simulink model "FordFocus2013_DirectDrive_2016a"  (R2016a)
settings: Solver=FixedStepAuto  SolverMode=SingleTasking  StartTime=0.0  StopTime=len  FixedStep=1e-3  RelTol=1e-3
values from neighbouring files (symbols this model uses):
  logvars = 4    [runFocusValidation_WindsorMotor_DirectDrive.m]
undefined symbols (not defined in the file or in its folder): accessory_load, chassis, driver, enviro, ess, fd, motor, veh_init_speed, wheel
libraries: simulink x2
settings Model: SimulationMode=accelerator  Creator=leahe  LastModifiedBy=chris
settings SolverCC: ZeroCrossAlgorithm=Adaptive
settings DataIOCC: LimitDataPoints=on  SaveFormat=Array
settings OptimizationCC: BlockReduction=off  BooleanDataType=off  EfficientMapNaN2IntZero=off
settings DebuggingCC: SaveWithParameterizedLinksMsg=none  UnderspecifiedInitializationDetection=Classic  MergeDetectMultiDrivingBlocksExec=none  SignalResolutionControl=TryResolveAllWithWarning
settings HardwareCC: ProdBitPerPointer=32  ProdLargestAtomicFloat=None  ProdIntDivRoundTo=Undefined  ProdEndianess=Unspecified  ProdWordSize=32  ProdHWDeviceType=32-bit Generic  TargetBitPerPointer=64  TargetLongLongMode=on  TargetIntDivRoundTo=Zero  TargetEndianess=LittleEndian  TargetWordSize=64  TargetHWDeviceType=MATLAB Host  ProdEqTarget=off
settings ModelReferenceCC: PropagateSignalLabelsOutOfModel=off
settings CodeAppCC: MaxIdLength=128
settings GRTTargetCC: GeneratePreprocessorConditionals=Use local settings  CombineOutputUpdateFcns=off  GRTInterface=on
settings ConfigComp: CovSFcnEnable=off

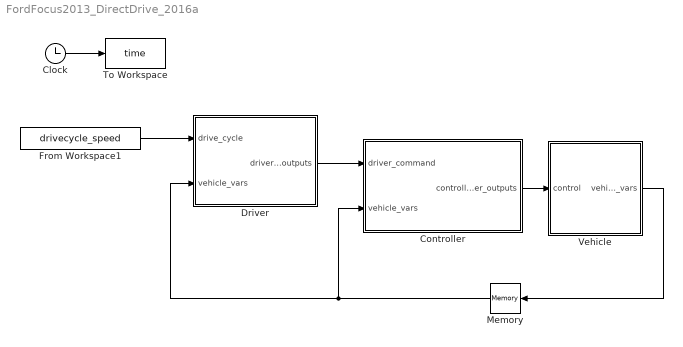
== system FordFocus2013_DirectDrive_2016a ==
  Clock : Clock
  Controller : Subsystem
  Driver : Subsystem
  From Workspace1 : FromWorkspace  VariableName=drivecycle_speed  SampleTime=0
  Memory : Memory
  To Workspace : ToWorkspace  VariableName=time  SampleTime=-1
      settings: Decimation=dec
  Vehicle : Subsystem
  wires:
  From Workspace1/1 -> Driver/1(drive_cycle)
  Memory/1 -> Driver/2(vehicle_vars), Controller/2(vehicle_vars)
  Controller/1(controller_outputs) -> Vehicle/1(control)
  Driver/1(driver_outputs) -> Controller/1(driver_command)
  Vehicle/1(vehicle_vars) -> Memory/1
  Clock/1 -> To Workspace/1

== system FordFocus2013_DirectDrive_2016a/Controller ==
  driver_command : Inport
  vehicle_vars : Inport  Port=2
  Bus Creator : BusCreator  Inputs=2
  Bus Selector : BusSelector  OutputSignals=trq_accel_dmd,trq_brk_dmd
  Bus Selector1 : BusSelector  OutputSignals=mot.mot_w,chas,ess1.ess_plant_volt_out
  Control Logic : Subsystem
  controller_outputs : Outport
  wires:
  driver_command/1 -> Bus Selector/1
  vehicle_vars/1 -> Bus Selector1/1
  Bus Creator/1 -> controller_outputs/1
  Bus Selector/1 -> Control Logic/1(driver_acceleration_cmd)  "<trq_accel_dmd>"
  Bus Selector/2 -> Control Logic/2(driver_brake_cmd)  "<trq_brk_dmd>"
  Control Logic/1(motor_trq_dmd) -> Bus Creator/1  "mot_trq_dmd"
  Control Logic/2(vehicle_wheel_dmd) -> Bus Creator/2  "whl_brk_trq_dmd"
  Bus Selector1/1 -> Control Logic/3(vehicle_motor_speed)  "<mot_w>"
  Bus Selector1/2 -> Control Logic/4(vehicle_chassis_speed)  "<chas>"
  Bus Selector1/3 -> Control Logic/5(ess2_voltage)  "<ess_plant_volt_out>"

== system FordFocus2013_DirectDrive_2016a/Driver ==
  drive_cycle : Inport
  vehicle_vars : Inport  Port=2
  Bus Creator1 : BusCreator  Inputs=3
  Bus Selector : BusSelector  OutputSignals=chas
  Plant : Subsystem
  Scope : Scope  NumInputPorts=2
  driver_outputs : Outport
  wires:
  drive_cycle/1 -> Scope/1, Plant/1(drive_cycle)
  Plant/1(driver_speed_dmd) -> Bus Creator1/1  "drv_lin_spd_dmd"
  vehicle_vars/1 -> Bus Selector/1
  Bus Selector/1 -> Scope/2, Plant/2(chassis_speed)  "<chas>"
  Bus Creator1/1 -> driver_outputs/1
  Plant/2(motor_torque_dmd) -> Bus Creator1/2  "trq_accel_dmd"
  Plant/3(wheel_brake_dmd) -> Bus Creator1/3  "trq_brk_dmd"

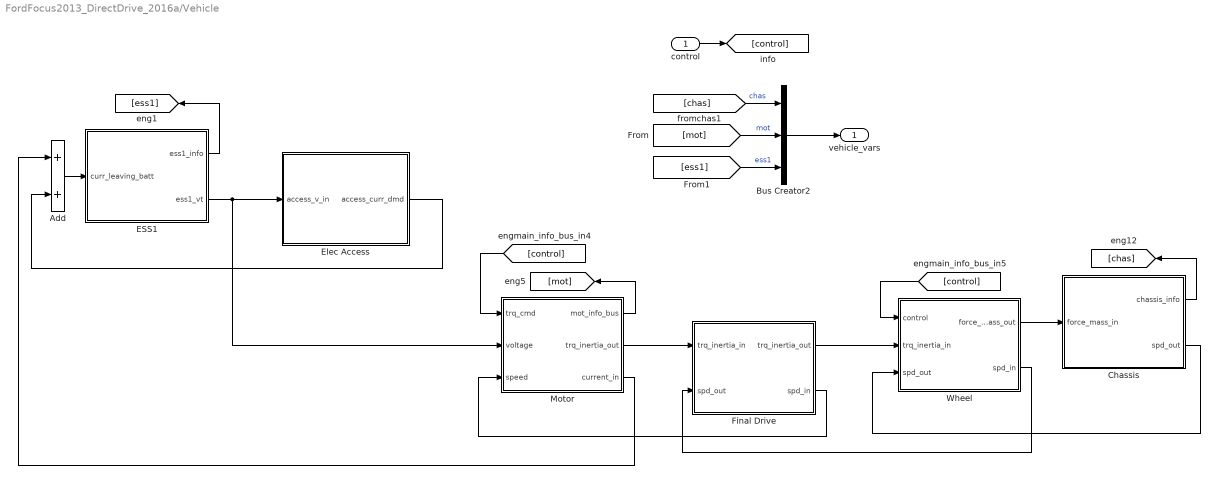
== system FordFocus2013_DirectDrive_2016a/Vehicle ==
  control : Inport
  Add : Sum
  Bus Creator2 : BusCreator  Inputs=3
  Chassis : Subsystem
  ESS1 : Subsystem
  Elec Access : Subsystem
  Final Drive : Subsystem
  Motor : Subsystem
  Wheel : Subsystem
  vehicle_vars : Outport
  wires:
  control/1 -> [control]
  Wheel/1(force_mass_out) -> Chassis/1(force_mass_in)
  Wheel/2(spd_in) -> Final Drive/2(spd_out)
  Chassis/2(spd_out) -> Wheel/3(spd_out)
  Final Drive/1(trq_inertia_out) -> Wheel/2(trq_inertia_in)
  [control] -> Wheel/1(control)
  Chassis/1(chassis_info) -> [chas]
  Bus Creator2/1 -> vehicle_vars/1
  [control] -> Motor/1(trq_cmd)
  Motor/2(trq_inertia_out) -> Final Drive/1(trq_inertia_in)
  Final Drive/2(spd_in) -> Motor/3(speed)
  Motor/1(mot_info_bus) -> [mot]
  Motor/3(current_in) -> Add/1
  [chas] -> Bus Creator2/1  "chas"
  [mot] -> Bus Creator2/2  "mot"
  Elec Access/1(access_curr_dmd) -> Add/2
  ESS1/2(ess1_vt) -> Motor/2(voltage), Elec Access/1(access_v_in)
  Add/1 -> ESS1/1(curr_leaving_batt)
  ESS1/1(ess1_info) -> [ess1]
  [ess1] -> Bus Creator2/3  "ess1"

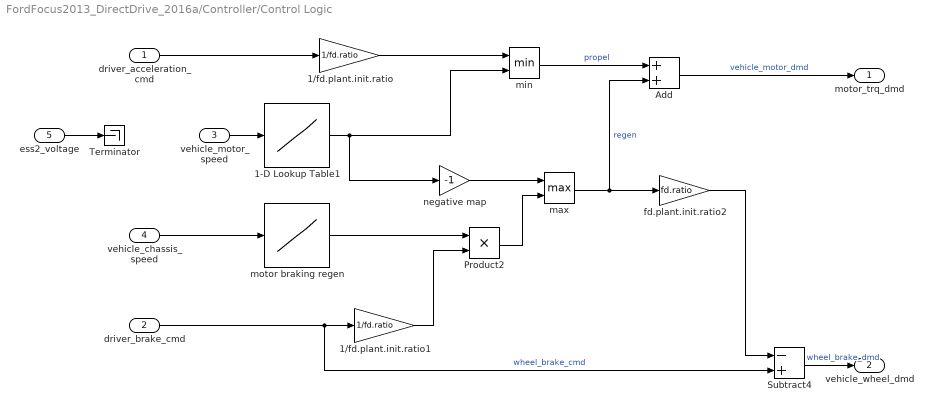
== system FordFocus2013_DirectDrive_2016a/Controller/Control Logic ==
  driver_acceleration_cmd : Inport
  driver_brake_cmd : Inport  Port=2
  vehicle_motor_speed : Inport  Port=3
  vehicle_chassis_speed : Inport  Port=4
  ess2_voltage : Inport  Port=5
  1-D Lookup Table1 : Lookup_n-D  NumberOfTableDimensions=1  BreakpointsForDimension1=motor.torquespeed_RPMidx  BreakpointsForDimension2=motor.torquespeed_RPMidx  IndexSearchMethod=Linear search  Table=motor.torquespeed_curveTOT  ExtrapMethod=Clip  UseLastTableValue=on  InternalRulePriority=Speed  RndMeth=Simplest  InputSameDT=on
  1/fd.plant.init.ratio : Gain  Gain=1/fd.ratio  SaturateOnIntegerOverflow=on  OutDataTypeStr=Inherit: Same as input  ParamDataTypeStr=Inherit: Same as input
  1/fd.plant.init.ratio1 : Gain  Gain=1/fd.ratio  SaturateOnIntegerOverflow=on  OutDataTypeStr=Inherit: Same as input  ParamDataTypeStr=Inherit: Same as input
  Add : Sum
  Product2 : Product
  Subtract4 : Sum  Inputs=-+
  Terminator : Terminator
  fd.plant.init.ratio2 : Gain  Gain=fd.ratio  SaturateOnIntegerOverflow=on  OutDataTypeStr=Inherit: Same as input  ParamDataTypeStr=Inherit: Same as input
  max : MinMax  Function=max  Inputs=2
  min : MinMax  Inputs=2
  motor braking regen : Lookup_n-D  NumberOfTableDimensions=1  BreakpointsForDimension1=motor.brake_idx  Table=motor.brake_map  InternalRulePriority=Speed  RndMeth=Simplest  InputSameDT=on
  negative map : Gain  Gain=-1  SaturateOnIntegerOverflow=on  OutDataTypeStr=Inherit: Same as input  ParamDataTypeStr=Inherit: Same as input
  motor_trq_dmd : Outport
  vehicle_wheel_dmd : Outport  Port=2
  wires:
  1/fd.plant.init.ratio/1 -> min/1
  1/fd.plant.init.ratio1/1 -> Product2/2
  Subtract4/1 -> vehicle_wheel_dmd/1  "wheel_brake_dmd"
  vehicle_chassis_speed/1 -> motor braking regen/1
  Product2/1 -> max/2
  vehicle_motor_speed/1 -> 1-D Lookup Table1/1
  driver_brake_cmd/1 -> Subtract4/2, 1/fd.plant.init.ratio1/1  "wheel_brake_cmd"
  driver_acceleration_cmd/1 -> 1/fd.plant.init.ratio/1
  min/1 -> Add/1  "propel"
  Add/1 -> motor_trq_dmd/1  "vehicle_motor_dmd"
  motor braking regen/1 -> Product2/1
  fd.plant.init.ratio2/1 -> Subtract4/1
  max/1 -> fd.plant.init.ratio2/1, Add/2  "regen"
  1-D Lookup Table1/1 -> negative map/1, min/2
  negative map/1 -> max/1
  ess2_voltage/1 -> Terminator/1

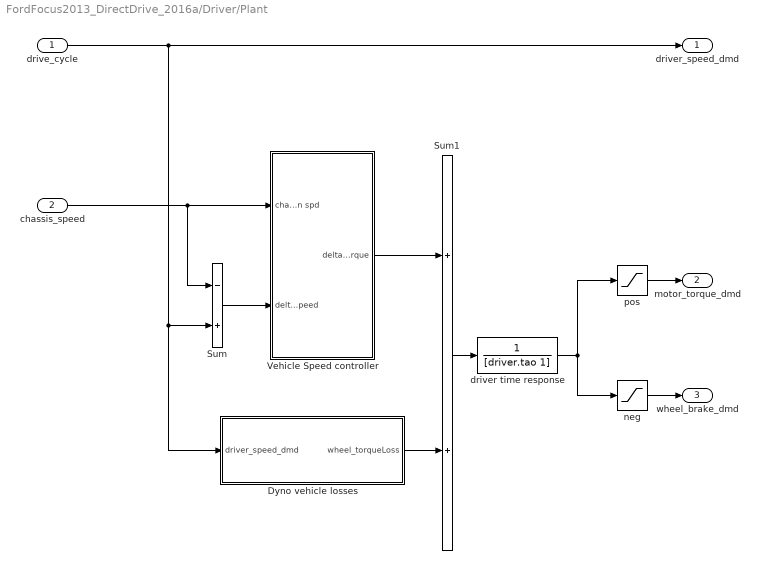
== system FordFocus2013_DirectDrive_2016a/Driver/Plant ==
  drive_cycle : Inport
  chassis_speed : Inport  Port=2
  Dyno vehicle losses : Subsystem
  Sum : Sum  Inputs=-+  SaturateOnIntegerOverflow=on  InputSameDT=on  OutDataTypeStr=Inherit: Same as first input
  Sum1 : Sum  Inputs=2  SaturateOnIntegerOverflow=on  InputSameDT=on  OutDataTypeStr=Inherit: Same as first input
  Vehicle Speed controller : Subsystem
  driver time response : TransferFcn  Denominator=[driver.tao 1]
  neg : Saturate  UpperLimit=0  LowerLimit=-inf
  pos : Saturate  UpperLimit=inf  LowerLimit=0
  driver_speed_dmd : Outport
  motor_torque_dmd : Outport  Port=2
  wheel_brake_dmd : Outport  Port=3
  wires:
  Vehicle Speed controller/1(delta torque) -> Sum1/1
  Dyno vehicle losses/1(wheel_torqueLoss) -> Sum1/2
  Sum/1 -> Vehicle Speed controller/2(delta speed)
  pos/1 -> motor_torque_dmd/1
  Sum1/1 -> driver time response/1
  neg/1 -> wheel_brake_dmd/1
  chassis_speed/1 -> Sum/1, Vehicle Speed controller/1(chas_lin spd)
  drive_cycle/1 -> Dyno vehicle losses/1(driver_speed_dmd), Sum/2, driver_speed_dmd/1
  driver time response/1 -> neg/1, pos/1

== system FordFocus2013_DirectDrive_2016a/Vehicle/Chassis ==
  force_mass_in : Inport
  From Workspace1 : FromWorkspace  VariableName=drivecycle_grade  SampleTime=0
  To Workspace : ToWorkspace  VariableName=chassis_speed  SampleTime=-1
      settings: Decimation=dec  Save2DSignal=2-D array (concatenate along first dimension)
  plant : Subsystem
  chassis_info : Outport
  spd_out : Outport  Port=2
  wires:
  plant/1(chas_lin_spd) -> spd_out/1, To Workspace/1, chassis_info/1
  force_mass_in/1 -> plant/2(chas_force_in chas_mass_in)
  From Workspace1/1 -> plant/1(Road grade)

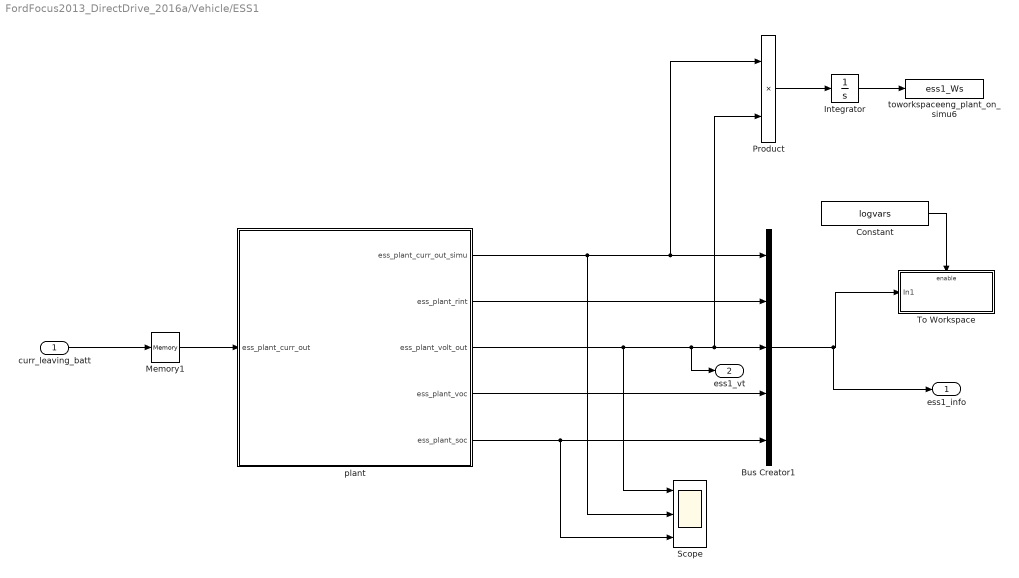
== system FordFocus2013_DirectDrive_2016a/Vehicle/ESS1 ==
  curr_leaving_batt : Inport
  Bus Creator1 : BusCreator  Inputs=5
  Constant : Constant  Value=logvars
  Integrator : Integrator
  Memory1 : Memory
  Product : Product
  Scope : Scope  NumInputPorts=3
  To Workspace : Subsystem  TreatAsAtomicUnit=on
  plant : Subsystem
  toworkspaceeng_plant_on_simu6 : ToWorkspace  VariableName=ess1_Ws  SampleTime=-1
      settings: Save2DSignal=2-D array (concatenate along first dimension)
  ess1_info : Outport
  ess1_vt : Outport  Port=2
  wires:
  Constant/1 -> To Workspace/Enable
  plant/4(ess_plant_voc) -> Bus Creator1/4
  plant/2(ess_plant_rint) -> Bus Creator1/2
  plant/1(ess_plant_curr_out_simu) -> Scope/2, Product/1, Bus Creator1/1
  curr_leaving_batt/1 -> Memory1/1
  Bus Creator1/1 -> ess1_info/1, To Workspace/1(In1)
  Memory1/1 -> plant/1(ess_plant_curr_out)
  plant/5(ess_plant_soc) -> Scope/3, Bus Creator1/5
  Product/1 -> Integrator/1
  Integrator/1 -> toworkspaceeng_plant_on_simu6/1
  plant/3(ess_plant_volt_out) -> Scope/1, ess1_vt/1, Product/2, Bus Creator1/3

== system FordFocus2013_DirectDrive_2016a/Vehicle/Elec Access ==
  access_v_in : Inport
  Electrical Power : Constant  Value=accessory_load
  Product : Product  Inputs=*/  SaturateOnIntegerOverflow=on  InputSameDT=on  OutDataTypeStr=Inherit: Same as first input
  Sum1 : Sum  SaturateOnIntegerOverflow=on  InputSameDT=on  OutDataTypeStr=Inherit: Same as first input
  eps : Constant  Value=eps
  access_curr_dmd : Outport
  wires:
  access_v_in/1 -> Sum1/1
  eps/1 -> Sum1/2
  Sum1/1 -> Product/2
  Electrical Power/1 -> Product/1
  Product/1 -> access_curr_dmd/1

== system FordFocus2013_DirectDrive_2016a/Vehicle/Final Drive ==
  trq_inertia_in : Inport
  spd_out : Inport  Port=2
  plant : Subsystem
  trq_inertia_out : Outport
  spd_in : Outport  Port=2
  wires:
  spd_out/1 -> plant/2(spd out)
  trq_inertia_in/1 -> plant/1(trq_inertia_in)
  plant/1(fd_trq_inertia_out) -> trq_inertia_out/1
  plant/2(fd_spd_in) -> spd_in/1

== system FordFocus2013_DirectDrive_2016a/Vehicle/Motor ==
  trq_cmd : Inport
  voltage : Inport  Port=2
  speed : Inport  Port=3
  Bus Creator : BusCreator  Inputs=3
  Bus Selector : BusSelector  OutputSignals=mot_trq_dmd
  motor : Subsystem
  mot_info_bus : Outport
  trq_inertia_out : Outport  Port=2
  current_in : Outport  Port=3
  wires:
  trq_cmd/1 -> Bus Selector/1
  voltage/1 -> motor/2(voltage)
  speed/1 -> motor/3(spd)
  motor/2(mot_current_in) -> Bus Creator/2, current_in/1
  motor/1(mot_trq_out mot_inertia_out) -> trq_inertia_out/1
  Bus Selector/1 -> motor/1(command_Nm)  "<mot_trq_dmd>"
  Bus Creator/1 -> mot_info_bus/1
  motor/4(motor_v_in) -> Bus Creator/3
  motor/3("speed out ") -> Bus Creator/1

== system FordFocus2013_DirectDrive_2016a/Vehicle/Wheel ==
  control : Inport
  trq_inertia_in : Inport  Port=2
  spd_out : Inport  Port=3
  Bus Selector : BusSelector  OutputSignals=whl_brk_trq_dmd
  From Workspace1 : FromWorkspace  VariableName=drivecycle_grade  SampleTime=0
  plant : Subsystem
  force_mass_out : Outport
  spd_in : Outport  Port=2
  wires:
  spd_out/1 -> plant/4(whl_spd)
  trq_inertia_in/1 -> plant/3(whl_trq_in whl_inertia_in)
  plant/2(whl_spd_in) -> spd_in/1
  plant/1(whl_force_out whl_mass_out) -> force_mass_out/1
  From Workspace1/1 -> plant/2(grade)
  control/1 -> Bus Selector/1
  Bus Selector/1 -> plant/1(brake trq dmd)  "<whl_brk_trq_dmd>"

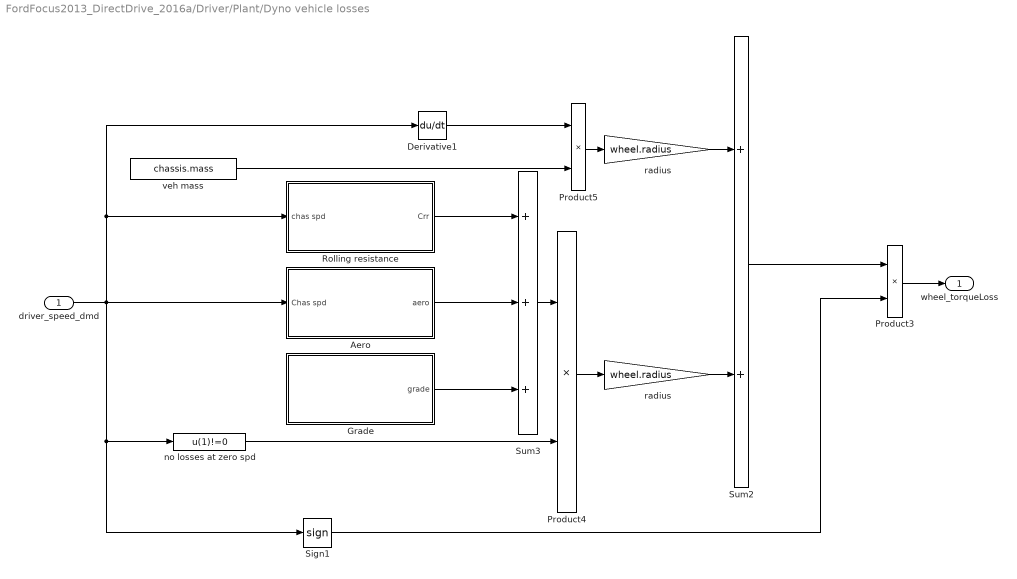
== system FordFocus2013_DirectDrive_2016a/Driver/Plant/Dyno vehicle losses ==
  driver_speed_dmd : Inport
  Aero : Subsystem
  Derivative1 : Derivative
  Grade : Subsystem
  Product3 : Product  SaturateOnIntegerOverflow=on  InputSameDT=on  OutDataTypeStr=Inherit: Same as first input
  Product4 : Product  SaturateOnIntegerOverflow=on  InputSameDT=on  OutDataTypeStr=Inherit: Same as first input
  Product5 : Product  SaturateOnIntegerOverflow=on  InputSameDT=on  OutDataTypeStr=Inherit: Same as first input
  Rolling resistance : Subsystem
  Sign1 : Signum
  Sum2 : Sum  Inputs=2  SaturateOnIntegerOverflow=on  InputSameDT=on  OutDataTypeStr=Inherit: Same as first input
  Sum3 : Sum  Inputs=3  SaturateOnIntegerOverflow=on  InputSameDT=on  OutDataTypeStr=Inherit: Same as first input
  no losses at zero spd : Fcn  Expr=u(1)!=0
  radius : Gain  Gain=wheel.radius  SaturateOnIntegerOverflow=on  OutDataTypeStr=Inherit: Same as input  ParamDataTypeStr=Inherit: Same as input
  "radius " : Gain  Gain=wheel.radius  SaturateOnIntegerOverflow=on  OutDataTypeStr=Inherit: Same as input  ParamDataTypeStr=Inherit: Same as input
  veh mass : Constant  Value=chassis.mass
  wheel_torqueLoss : Outport
  wires:
  "radius "/1 -> Sum2/2
  radius/1 -> Sum2/1
  no losses at zero spd/1 -> Product4/2
  Sum3/1 -> Product4/1
  Sign1/1 -> Product3/2
  veh mass/1 -> Product5/2
  Derivative1/1 -> Product5/1
  Product3/1 -> wheel_torqueLoss/1
  Sum2/1 -> Product3/1
  Product4/1 -> "radius "/1
  Product5/1 -> radius/1
  driver_speed_dmd/1 -> Sign1/1, no losses at zero spd/1, Aero/1(Chas spd), Derivative1/1, Rolling resistance/1(chas spd)
  Grade/1(grade) -> Sum3/3
  Aero/1(aero) -> Sum3/2
  Rolling resistance/1(Crr) -> Sum3/1

== system FordFocus2013_DirectDrive_2016a/Driver/Plant/Vehicle Speed controller ==
  chas_lin spd : Inport
  delta speed : Inport  Port=2  OutDataTypeStr=double
  "  1" : RelationalOperator  Operator=<  InputSameDT=on
  PID Controller : simulink/Continuous/PID Controller  Controller=PID  TimeDomain=Continuous-time  SampleTime=-1  IntegratorMethod=Forward Euler  FilterMethod=Forward Euler  Form=Parallel  UseFilter=on  ControllerParametersSource=internal  P=driver.p  I=driver.i  D=0  N=100  InitialConditionSource=internal  InitialConditionForIntegrator=0  InitialConditionForFilter=0  ExternalReset=either  LimitOutput=off  UpperSaturationLimit=inf  LowerSaturationLimit=-inf  LinearizeAsGain=on  AntiWindupMode=none  Kb=1  TrackingMode=off  Kt=1  PParamMin=[]  PParamMax=[]  IParamMin=[]  IParamMax=[]  DParamMin=[]  DParamMax=[]  NParamMin=[]  NParamMax=[]  KbParamMin=[]  KbParamMax=[]  KtParamMin=[]  KtParamMax=[]  POutMin=[]  POutMax=[]  IOutMin=[]  IOutMax=[]  DOutMin=[]  DOutMax=[]  NOutMin=[]  NOutMax=[]  KbOutMin=[]  KbOutMax=[]  KtOutMin=[]  KtOutMax=[]  IntegratorOutMin=[]  IntegratorOutMax=[]  FilterOutMin=[]  FilterOutMax=[]  SumOutMin=[]  SumOutMax=[]  SumI1OutMin=[]  SumI1OutMax=[]  SumI2OutMin=[]  SumI2OutMax=[]  SumI3OutMin=[]  SumI3OutMax=[]  SumDOutMin=[]  SumDOutMax=[]  SaturationOutMin=[]  SaturationOutMax=[]  IntegratorContinuousStateAttributes=''  IntegratorStateMustResolveToSignalObject=off  IntegratorRTWStateStorageClass=Auto  FilterContinuousStateAttributes=''  FilterStateMustResolveToSignalObject=off  FilterRTWStateStorageClass=Auto  DifferentiatorICPrevScaledInput=0  DifferentiatorOutMin=[]  DifferentiatorOutMax=[]
  "lin_spd_below_which_chas_stopped " : Constant  Value=driver.carStopped
  delta torque : Outport
  wires:
  PID Controller/1 -> delta torque/1
  chas_lin spd/1 -> "  1"/1
  "lin_spd_below_which_chas_stopped "/1 -> "  1"/2
  delta speed/1 -> PID Controller/1
  "  1"/1 -> PID Controller/2

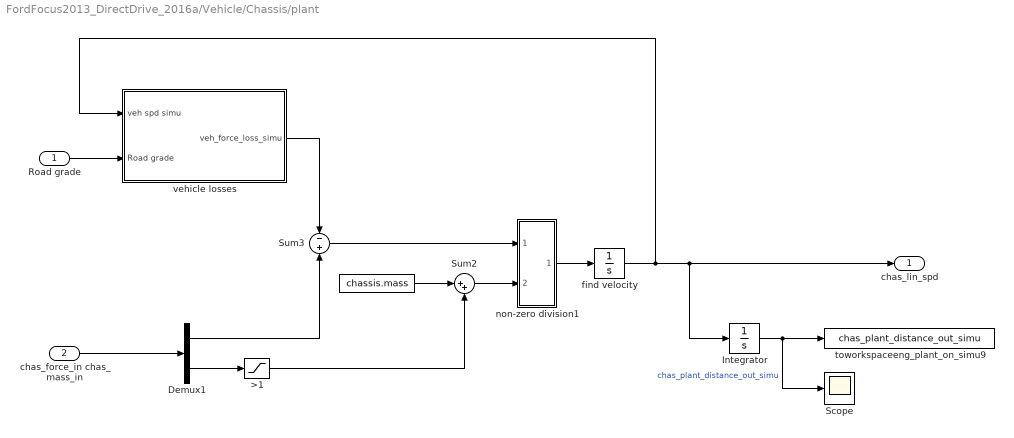
== system FordFocus2013_DirectDrive_2016a/Vehicle/Chassis/plant ==
  Road grade : Inport
  chas_force_in chas_mass_in : Inport  Port=2
  " " : Constant  Value=chassis.mass
  >1 : Saturate  UpperLimit=inf  LowerLimit=0
  Demux1 : Demux  Outputs=2
  Integrator : Integrator
  Scope : Scope
  Sum2 : Sum  Inputs=|++  SaturateOnIntegerOverflow=on  InputSameDT=on  OutDataTypeStr=Inherit: Same as first input
  Sum3 : Sum  Inputs=-+  SaturateOnIntegerOverflow=on  InputSameDT=on  OutDataTypeStr=Inherit: Same as first input
  find velocity : Integrator  InitialCondition=veh_init_speed  LimitOutput=on  LowerSaturationLimit=0
  non-zero division1 : Subsystem
      mask Display: disp('divider \n I1/I2')
  toworkspaceeng_plant_on_simu9 : ToWorkspace  VariableName=chas_plant_distance_out_simu  SampleTime=-1
      settings: Decimation=dec
  vehicle losses : Subsystem
  chas_lin_spd : Outport
  wires:
  Integrator/1 -> Scope/1, toworkspaceeng_plant_on_simu9/1  "chas_plant_distance_out_simu"
  " "/1 -> Sum2/1
  Road grade/1 -> vehicle losses/2(Road grade)
  find velocity/1 -> vehicle losses/1(veh spd simu), chas_lin_spd/1, Integrator/1
  non-zero division1/1(Out1) -> find velocity/1
  Sum3/1 -> non-zero division1/1(In1)
  Sum2/1 -> non-zero division1/2(In2)
  >1/1 -> Sum2/2
  Demux1/2 -> >1/1
  Demux1/1 -> Sum3/2
  chas_force_in chas_mass_in/1 -> Demux1/1
  vehicle losses/1(veh_force_loss_simu) -> Sum3/1

== system FordFocus2013_DirectDrive_2016a/Vehicle/ESS1/To Workspace ==
  In1 : Inport
  Enable : EnablePort
  Bus Selector : BusSelector  OutputSignals=ess_plant_curr_simu,ess_plant_rint,ess_plant_volt_out,ess_plant_voc,ess_plant_soc
  toworkspaceeng_plant_on_simu1 : ToWorkspace  VariableName=ess_i  SampleTime=-1
      settings: Decimation=dec
  toworkspaceeng_plant_on_simu2 : ToWorkspace  VariableName=ess_rint  SampleTime=-1
      settings: Decimation=dec
  toworkspaceeng_plant_on_simu3 : ToWorkspace  VariableName=ess_v  SampleTime=-1
      settings: Decimation=dec
  toworkspaceeng_plant_on_simu4 : ToWorkspace  VariableName=ess_voc  SampleTime=-1
      settings: Decimation=dec
  toworkspaceeng_plant_on_simu5 : ToWorkspace  VariableName=ess_soc  SampleTime=-1
      settings: Decimation=dec
  wires:
  Bus Selector/5 -> toworkspaceeng_plant_on_simu5/1  "<ess_plant_soc>"
  Bus Selector/4 -> toworkspaceeng_plant_on_simu4/1  "<ess_plant_voc>"
  Bus Selector/3 -> toworkspaceeng_plant_on_simu3/1  "<ess_plant_volt_out>"
  Bus Selector/2 -> toworkspaceeng_plant_on_simu2/1  "<ess_plant_rint>"
  Bus Selector/1 -> toworkspaceeng_plant_on_simu1/1  "<ess_plant_curr_simu>"
  In1/1 -> Bus Selector/1

== system FordFocus2013_DirectDrive_2016a/Vehicle/ESS1/plant ==
  ess_plant_curr_out : Inport
  Relational Operator : RelationalOperator  Operator=<  OutDataTypeStr=boolean
  Stop Simulation : Stop
  ess_plant_soc_calculation : Subsystem
  ess_plant_volt_calculation : Subsystem
  soc_min : Constant  Value=ess.soc_min
  ess_plant_curr_out_simu : Outport
  ess_plant_rint : Outport  Port=2
  ess_plant_volt_out : Outport  Port=3
  ess_plant_voc : Outport  Port=4
  ess_plant_soc : Outport  Port=5
  wires:
  ess_plant_curr_out/1 -> ess_plant_soc_calculation/1(ess_plant_curr_out), ess_plant_volt_calculation/2(Current), ess_plant_curr_out_simu/1  "ess_plant_curr_simu"
  ess_plant_volt_calculation/3(Rint) -> ess_plant_rint/1  "ess_plant_rint"
  ess_plant_volt_calculation/1(Voc) -> ess_plant_voc/1  "ess_plant_voc"
  ess_plant_volt_calculation/2(volt) -> ess_plant_volt_out/1  "ess_plant_volt_out"
  ess_plant_soc_calculation/1(ess_plant_soc) -> ess_plant_volt_calculation/1(SOC (prev)), Relational Operator/1, ess_plant_soc/1  "ess_plant_soc"
  soc_min/1 -> Relational Operator/2
  Relational Operator/1 -> Stop Simulation/1

== system FordFocus2013_DirectDrive_2016a/Vehicle/Final Drive/plant ==
  trq_inertia_in : Inport
  spd out : Inport  Port=2
  Demux : Demux  Outputs=2
  Inertia calculation : Subsystem
  Mux1 : Mux  Inputs=2
  Speed calculation : Subsystem
  Torque calculation : Subsystem
  fd_trq_inertia_out : Outport
  fd_spd_in : Outport  Port=2
  wires:
  spd out/1 -> Speed calculation/1(spd out)
  Torque calculation/1(trq out) -> Mux1/1  "fd_trq_out_simu"
  Demux/1 -> Torque calculation/2(trq in)
  Inertia calculation/1(inertia out) -> Mux1/2  "fd_inertia_out_simu"
  Demux/2 -> Inertia calculation/1(inertia in)
  Speed calculation/1(spd in) -> Torque calculation/1(spd in), fd_spd_in/1
  Mux1/1 -> fd_trq_inertia_out/1
  trq_inertia_in/1 -> Demux/1

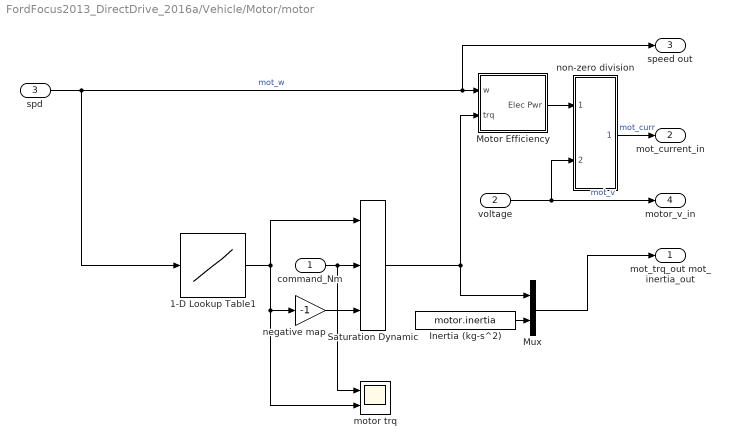
== system FordFocus2013_DirectDrive_2016a/Vehicle/Motor/motor ==
  command_Nm : Inport
  voltage : Inport  Port=2
  spd : Inport  Port=3
  1-D Lookup Table1 : Lookup_n-D  NumberOfTableDimensions=1  BreakpointsForDimension1=motor.torquespeed_RPMidx  BreakpointsForDimension2=motor.torquespeed_RPMidx  IndexSearchMethod=Linear search  Table=motor.torquespeed_curveTOT  ExtrapMethod=Clip  UseLastTableValue=on  InternalRulePriority=Speed  RndMeth=Simplest  InputSameDT=on
  Inertia (kg-s^2) : Constant  Value=motor.inertia
  Motor Efficiency : Subsystem
  Mux : Mux  Inputs=2
  Saturation Dynamic : simulink/Discontinuities/Saturation Dynamic  OutMin=[]  OutMax=[]  OutDataTypeStr=Inherit: Same as second input  OutDataType=fixdt(1, 16)  OutScaling=2^-10  DoSatur=off
  motor trq : Scope  NumInputPorts=2
  negative map : Gain  Gain=-1
  non-zero division : Subsystem
      mask Display: disp('divider \n I1/I2')
  mot_trq_out mot_inertia_out : Outport
  mot_current_in : Outport  Port=2
  "speed out " : Outport  Port=3
  motor_v_in : Outport  Port=4
  wires:
  non-zero division/1(Out1) -> mot_current_in/1  "mot_curr"
  Mux/1 -> mot_trq_out mot_inertia_out/1
  Inertia (kg-s^2)/1 -> Mux/2
  Saturation Dynamic/1 -> Motor Efficiency/2(trq), Mux/1
  Motor Efficiency/1(Elec Pwr) -> non-zero division/1(In1)
  negative map/1 -> Saturation Dynamic/3
  command_Nm/1 -> Saturation Dynamic/2, motor trq/1
  spd/1 -> 1-D Lookup Table1/1, "speed out "/1, Motor Efficiency/1(w)  "mot_w"
  1-D Lookup Table1/1 -> motor trq/2, negative map/1, Saturation Dynamic/1
  voltage/1 -> non-zero division/2(In2), motor_v_in/1  "mot_v"

== system FordFocus2013_DirectDrive_2016a/Vehicle/Wheel/plant ==
  brake trq dmd : Inport
  grade : Inport  Port=2
  whl_trq_in whl_inertia_in : Inport  Port=3
  whl_spd : Inport  Port=4
  "1\\radius " : Gain  Gain=1/wheel.radius  SaturateOnIntegerOverflow=on  OutDataTypeStr=Inherit: Same as input  ParamDataTypeStr=Inherit: Same as input
  Demux : Demux  Outputs=2
  Force calculation : Subsystem
  Mass calculation : Subsystem
  Mux1 : Mux  Inputs=2
  whl_force_out whl_mass_out : Outport
  whl_spd_in : Outport  Port=2
  wires:
  grade/1 -> Force calculation/2(grade)
  Mux1/1 -> whl_force_out whl_mass_out/1
  brake trq dmd/1 -> Force calculation/3(brake trq dmd)
  whl_trq_in whl_inertia_in/1 -> Demux/1
  whl_spd/1 -> Force calculation/1(whl_spd), "1\\radius "/1
  Demux/2 -> Mass calculation/1(inertia in)
  Demux/1 -> Force calculation/4(trq in)
  Mass calculation/1(Mass) -> Mux1/2  "whl_mass_out_simu"
  "1\\radius "/1 -> whl_spd_in/1
  Force calculation/1(force) -> Mux1/1  "whl_force_out_simu"

== system FordFocus2013_DirectDrive_2016a/Driver/Plant/Dyno vehicle losses/Aero ==
  Chas spd : Inport
  Gain : Gain  Gain=0.5
  Product2 : Product  Inputs=5  SaturateOnIntegerOverflow=on  InputSameDT=on  OutDataTypeStr=Inherit: Same as first input
  veh mass7 : Constant  Value=enviro.dens_air
  veh mass8 : Constant  Value=chassis.cd
  veh mass9 : Constant  Value=chassis.area
  aero : Outport
  wires:
  Product2/1 -> Gain/1
  veh mass7/1 -> Product2/3
  veh mass8/1 -> Product2/4
  veh mass9/1 -> Product2/5
  Chas spd/1 -> Product2/2, Product2/1
  Gain/1 -> aero/1  "Drag Force"

== system FordFocus2013_DirectDrive_2016a/Driver/Plant/Dyno vehicle losses/Grade ==
  From Workspace1 : FromWorkspace  VariableName=drivecycle_grade  SampleTime=0
  Product1 : Product  Inputs=3  SaturateOnIntegerOverflow=on  InputSameDT=on  OutDataTypeStr=Inherit: Same as first input
  Trigonometric Function1 : Trigonometry
  veh mass1 : Constant  Value=enviro.gravity
  veh mass2 : Constant  Value=chassis.mass
  grade : Outport
  wires:
  veh mass2/1 -> Product1/2
  From Workspace1/1 -> Trigonometric Function1/1
  Trigonometric Function1/1 -> Product1/1
  veh mass1/1 -> Product1/3
  Product1/1 -> grade/1  "Grade Force"

== system FordFocus2013_DirectDrive_2016a/Driver/Plant/Dyno vehicle losses/Rolling resistance ==
  chas spd : Inport
  From Workspace2 : FromWorkspace  VariableName=drivecycle_grade  SampleTime=0
  Product7 : Product  SaturateOnIntegerOverflow=on  InputSameDT=on  OutDataTypeStr=Inherit: Same as first input
  Product8 : Product  Inputs=4  SaturateOnIntegerOverflow=on  InputSameDT=on  OutDataTypeStr=Inherit: Same as first input
  Sum1 : Sum  Inputs=2  SaturateOnIntegerOverflow=on  InputSameDT=on  OutDataTypeStr=Inherit: Same as first input
  Trigonometric Function2 : Trigonometry  Operator=cos
  veh mass : Constant  Value=chassis.mass
  veh mass4 : Constant  Value=wheel.u2
  veh mass5 : Constant  Value=wheel.u1
  veh mass6 : Constant  Value=enviro.gravity
  Crr : Outport
  wires:
  From Workspace2/1 -> Trigonometric Function2/1
  veh mass4/1 -> Product7/2
  veh mass5/1 -> Sum1/2
  Product7/1 -> Sum1/1
  Sum1/1 -> Product8/2
  veh mass6/1 -> Product8/3
  Trigonometric Function2/1 -> Product8/1
  veh mass/1 -> Product8/4
  chas spd/1 -> Product7/1
  Product8/1 -> Crr/1  "Rolling resistance"

== system FordFocus2013_DirectDrive_2016a/Vehicle/Chassis/plant/non-zero division1 ==
  note: (u[2]==0) is true then returns 1, thus (u[2]+(u[2]==0)) is equal to 0+1=1
  note: if u[2] == 0, then output == 0:
  note: (u[2]!=0) is false then returns 0
  note: and finally, the expression is: (u[1] \ 1) * 0 = 0
  note: (u[2]==0) is false then returns 0, thus (u[2]+(u[2]==0)) is equal to u[2]+0=u[2]
  note: if u[2] != 0, then output == u[1]\u[2]:
  note: (u[2]!=0) is true then returns 1
  note: and finally, the expression is: (u[1] \ u[2]) * 1 = u[1] \ u[2]
  In1 : Inport
  In2 : Inport  Port=2
  Fcn : Fcn  Expr=u[1]/(u[2]+(u[2]==0))*(u[2]!=0)
  Mux : Mux  Inputs=2
  Out1 : Outport
  wires:
  Mux/1 -> Fcn/1
  In1/1 -> Mux/1
  Fcn/1 -> Out1/1
  In2/1 -> Mux/2

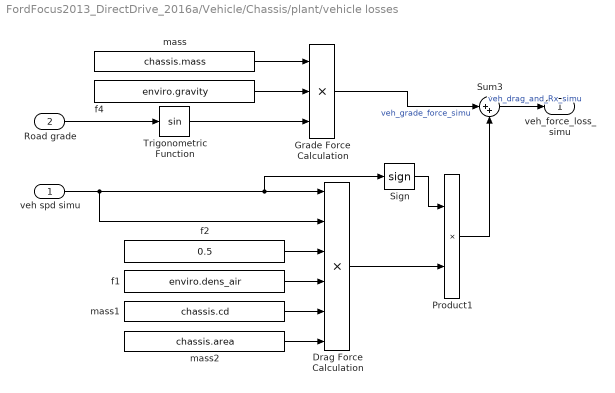
== system FordFocus2013_DirectDrive_2016a/Vehicle/Chassis/plant/vehicle losses ==
  veh spd simu : Inport
  Road grade : Inport  Port=2
  Drag Force Calculation : Product  Inputs=6  SaturateOnIntegerOverflow=on  InputSameDT=on  OutDataTypeStr=Inherit: Same as first input
  Grade Force Calculation : Product  Inputs=3  SaturateOnIntegerOverflow=on  InputSameDT=on  OutDataTypeStr=Inherit: Same as first input
  Product1 : Product  SaturateOnIntegerOverflow=on  InputSameDT=on  OutDataTypeStr=Inherit: Same as first input
  Sign : Signum
  Sum3 : Sum  Inputs=|++  SaturateOnIntegerOverflow=on  InputSameDT=on  OutDataTypeStr=Inherit: Same as first input
  Trigonometric Function : Trigonometry
  f1 : Constant  Value=enviro.dens_air
  f2 : Constant  Value=0.5
  f4 : Constant  Value=enviro.gravity
  mass : Constant  Value=chassis.mass
  mass1 : Constant  Value=chassis.cd
  mass2 : Constant  Value=chassis.area
  veh_force_loss_simu : Outport
  wires:
  f2/1 -> Drag Force Calculation/3
  mass2/1 -> Drag Force Calculation/6
  mass1/1 -> Drag Force Calculation/5
  f1/1 -> Drag Force Calculation/4
  Trigonometric Function/1 -> Grade Force Calculation/3
  f4/1 -> Grade Force Calculation/2
  mass/1 -> Grade Force Calculation/1
  Product1/1 -> Sum3/2
  Sign/1 -> Product1/1
  Road grade/1 -> Trigonometric Function/1
  Drag Force Calculation/1 -> Product1/2
  veh spd simu/1 -> Drag Force Calculation/1, Sign/1, Drag Force Calculation/2
  Grade Force Calculation/1 -> Sum3/1  "veh_grade_force_simu"
  Sum3/1 -> veh_force_loss_simu/1  "veh_drag_and_Rx_simu"

== system FordFocus2013_DirectDrive_2016a/Vehicle/ESS1/plant/ess_plant_soc_calculation ==
  ess_plant_curr_out : Inport
  (sec->hrs) : Gain  Gain=1/3600  SaturateOnIntegerOverflow=on  OutDataTypeStr=Inherit: Same as input  ParamDataTypeStr=Inherit: Same as input
  (sec->hrs)1 : Gain  Gain=-1  SaturateOnIntegerOverflow=on  OutDataTypeStr=Inherit: Same as input  ParamDataTypeStr=Inherit: Same as input
  Constant : Constant  Value=ess.soc_start
  Constant1 : Constant  Value=ess.cap
  Integrator : Integrator  InitialConditionSource=external
  Product : Product  RndMeth=Zero
  non-zero division1 : Subsystem
      mask Display: disp('divider \n I1/I2')
  ess_plant_soc : Outport
  wires:
  Constant1/1 -> non-zero division1/2(In2), Product/2
  non-zero division1/1(Out1) -> ess_plant_soc/1
  (sec->hrs)/1 -> (sec->hrs)1/1
  Integrator/1 -> non-zero division1/1(In1)
  Constant/1 -> Product/1
  Product/1 -> Integrator/2
  (sec->hrs)1/1 -> Integrator/1
  ess_plant_curr_out/1 -> (sec->hrs)/1

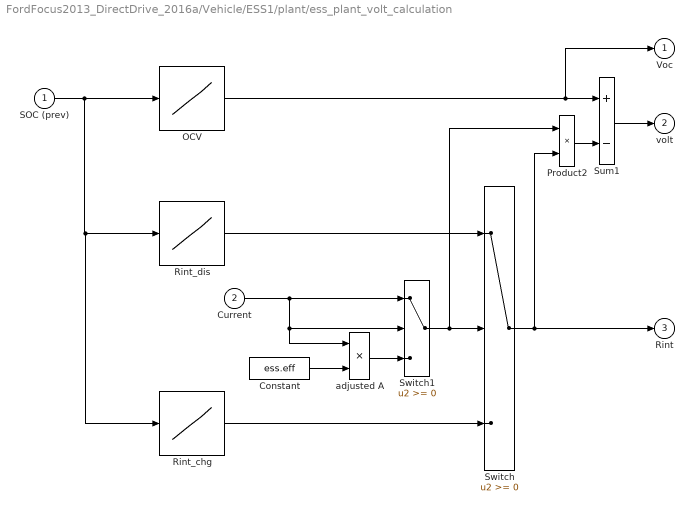
== system FordFocus2013_DirectDrive_2016a/Vehicle/ESS1/plant/ess_plant_volt_calculation ==
  SOC (prev) : Inport
  Current : Inport  Port=2
  Constant : Constant  Value=ess.eff
  OCV : Lookup_n-D  NumberOfTableDimensions=1  BreakpointsForDimension1=ess.idx_soc  BreakpointsForDimension2=ess.plant.init.voc.idx2_soc  Table=ess.ocv_map  ExtrapMethod=Clip  UseLastTableValue=on  RndMeth=Simplest  InputSameDT=on
  Product2 : Product  SaturateOnIntegerOverflow=on  InputSameDT=on  OutDataTypeStr=Inherit: Same as first input
  Rint_chg : Lookup_n-D  NumberOfTableDimensions=1  BreakpointsForDimension1=ess.rchg.idx_soc  BreakpointsForDimension2=ess.plant.init.rint_chg.idx2_soc  Table=ess.rchg_map  ExtrapMethod=Clip  UseLastTableValue=on  RndMeth=Simplest  InputSameDT=on
  Rint_dis : Lookup_n-D  NumberOfTableDimensions=1  BreakpointsForDimension1=ess.rdis.idx_soc  BreakpointsForDimension2=ess.plant.init.rint_dis.idx2_soc  Table=ess.rdis_map  ExtrapMethod=Clip  UseLastTableValue=on  RndMeth=Simplest  InputSameDT=on
  Sum1 : Sum  Inputs=+-  SaturateOnIntegerOverflow=on  InputSameDT=on  OutDataTypeStr=Inherit: Same as first input
  Switch : Switch  SaturateOnIntegerOverflow=on  InputSameDT=on
  Switch1 : Switch  SaturateOnIntegerOverflow=on  InputSameDT=on
  adjusted A : Product  SaturateOnIntegerOverflow=on  InputSameDT=on  OutDataTypeStr=Inherit: Same as first input
  Voc : Outport  InitialOutput=0
  volt : Outport  Port=2  InitialOutput=0
  Rint : Outport  Port=3  InitialOutput=0
  wires:
  Switch/1 -> Rint/1, Product2/2
  Switch1/1 -> Switch/2, Product2/1
  Rint_dis/1 -> Switch/1
  Rint_chg/1 -> Switch/3
  OCV/1 -> Sum1/1, Voc/1
  SOC (prev)/1 -> OCV/1, Rint_dis/1, Rint_chg/1
  Product2/1 -> Sum1/2
  Sum1/1 -> volt/1
  Constant/1 -> adjusted A/2
  Current/1 -> Switch1/1, Switch1/2, adjusted A/1
  adjusted A/1 -> Switch1/3

== system FordFocus2013_DirectDrive_2016a/Vehicle/Final Drive/plant/Inertia calculation ==
  inertia in : Inport
  " " : Constant  Value=fd.inert
  Sum3 : Sum  Inputs=|++  SaturateOnIntegerOverflow=on  InputSameDT=on  OutDataTypeStr=Inherit: Same as first input
  fd.plant.init.ratio : Gain  Gain=fd.ratio  SaturateOnIntegerOverflow=on  OutDataTypeStr=Inherit: Same as input  ParamDataTypeStr=Inherit: Same as input
  inertia out : Outport
  wires:
  inertia in/1 -> fd.plant.init.ratio/1
  fd.plant.init.ratio/1 -> Sum3/1
  " "/1 -> Sum3/2
  Sum3/1 -> inertia out/1

== system FordFocus2013_DirectDrive_2016a/Vehicle/Final Drive/plant/Speed calculation ==
  spd out : Inport
  " " : Gain  Gain=fd.ratio  SaturateOnIntegerOverflow=on  OutDataTypeStr=Inherit: Same as input  ParamDataTypeStr=Inherit: Same as input
  spd in : Outport
  wires:
  spd out/1 -> " "/1
  " "/1 -> spd in/1

== system FordFocus2013_DirectDrive_2016a/Vehicle/Final Drive/plant/Torque calculation ==
  spd in : Inport
  trq in : Inport  Port=2
  " " : Gain  Gain=fd.ratio  SaturateOnIntegerOverflow=on  OutDataTypeStr=Inherit: Same as input  ParamDataTypeStr=Inherit: Same as input
  Abs : Abs  SaturateOnIntegerOverflow=on
  Abs1 : Abs  SaturateOnIntegerOverflow=on
  Efficiency : Lookup_n-D  BreakpointsForDimension1=fd.torque  BreakpointsForDimension2=fd.speed  Table=fd.effmap  ExtrapMethod=Clip  UseLastTableValue=on  InternalRulePriority=Speed  RndMeth=Simplest  InputSameDT=on
  Product1 : Product
  Sign : Signum
  Switch : Switch  Criteria=u2 > Threshold
  non-zero division1 : Subsystem
      mask Display: disp('divider \n I1/I2')
  trq out : Outport
  wires:
  Abs/1 -> Efficiency/1
  Abs1/1 -> Efficiency/2
  spd in/1 -> Abs1/1
  trq in/1 -> Sign/1, " "/1, Abs/1
  " "/1 -> Product1/2, non-zero division1/1(In1)
  Sign/1 -> Switch/2
  Switch/1 -> trq out/1
  Efficiency/1 -> non-zero division1/2(In2), Product1/1
  Product1/1 -> Switch/1
  non-zero division1/1(Out1) -> Switch/3

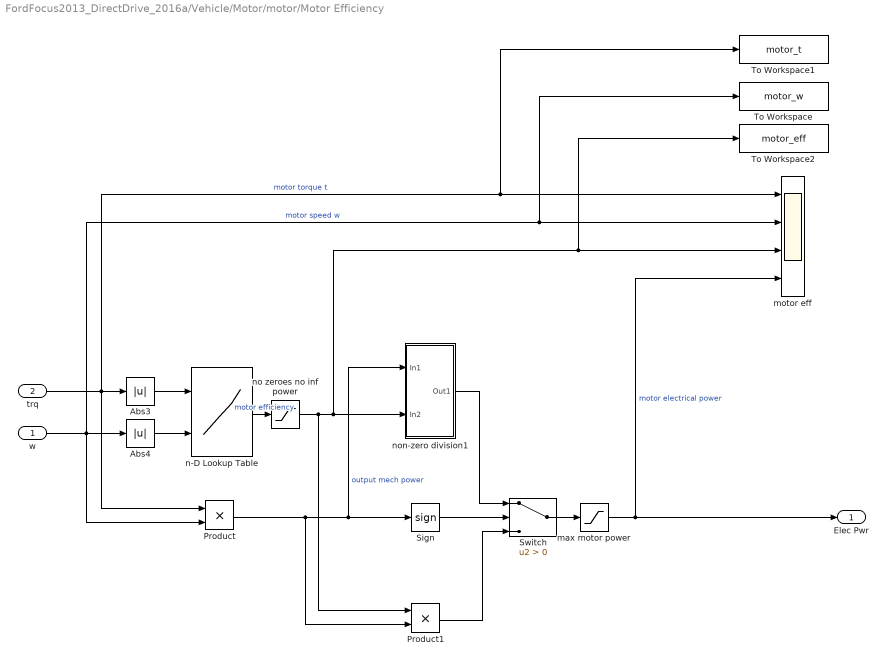
== system FordFocus2013_DirectDrive_2016a/Vehicle/Motor/motor/Motor Efficiency ==
  w : Inport
  trq : Inport  Port=2
  Abs3 : Abs
  Abs4 : Abs
  Product : Product
  Product1 : Product
  Sign : Signum
  Switch : Switch  Criteria=u2 > Threshold
  To Workspace : ToWorkspace  VariableName=motor_w  SampleTime=-1
      settings: Save2DSignal=2-D array (concatenate along first dimension)
  To Workspace1 : ToWorkspace  VariableName=motor_t  SampleTime=-1
      settings: Save2DSignal=2-D array (concatenate along first dimension)
  To Workspace2 : ToWorkspace  VariableName=motor_eff  SampleTime=-1
      settings: Save2DSignal=2-D array (concatenate along first dimension)
  max motor power : Saturate  UpperLimit=motor.prated  LowerLimit=-(motor.prated)  LinearizeAsGain=off
  motor eff : Scope  NumInputPorts=4
  n-D Lookup Table : Lookup_n-D  BreakpointsForDimension1=motor.spd_ind  BreakpointsForDimension2=motor.trq_ind  BreakpointsForDimension3=motor.vol_ind  IndexSearchMethod=Linear search  Table=motor.eff_map  ExtrapMethod=Clip  UseLastTableValue=on  InternalRulePriority=Speed  RndMeth=Simplest  InputSameDT=on
  no zeroes no inf power : Saturate  UpperLimit=1  LowerLimit=0.7  LinearizeAsGain=off
  non-zero division1 : Subsystem
      mask Display: disp('divider \n I1/I2')
  Elec Pwr : Outport
  wires:
  Sign/1 -> Switch/2
  non-zero division1/1(Out1) -> Switch/1
  Product1/1 -> Switch/3
  Product/1 -> Product1/2, non-zero division1/1(In1), Sign/1  "output mech power"
  Switch/1 -> max motor power/1
  max motor power/1 -> motor eff/4, Elec Pwr/1  "motor electrical power"
  w/1 -> Product/2, To Workspace/1, motor eff/2, Abs4/1  "motor speed w"
  trq/1 -> Product/1, motor eff/1, To Workspace1/1, Abs3/1  "motor torque t"
  n-D Lookup Table/1 -> no zeroes no inf power/1  "motor efficiency"
  Abs3/1 -> n-D Lookup Table/1
  Abs4/1 -> n-D Lookup Table/2
  no zeroes no inf power/1 -> Product1/1, To Workspace2/1, motor eff/3, non-zero division1/2(In2)

== system FordFocus2013_DirectDrive_2016a/Vehicle/Motor/motor/non-zero division ==
  note: original idea from Phil Sharer - ANL
      | original formula: u[1]\(u[2]+eps)*(u[2]!=0)
      | changes done by Gerald ZINI (dgey) - ANL (05\02\2001)
  note: (u[2]==0) is true then returns 1, thus (u[2]+(u[2]==0)) is equal to 0+1=1
  note: if u[2] == 0, then output == 0:
  note: (u[2]!=0) is false then returns 0
  note: and finally, the expression is: (u[1] \ 1) * 0 = 0
  note: (u[2]==0) is false then returns 0, thus (u[2]+(u[2]==0)) is equal to u[2]+0=u[2]
  note: if u[2] != 0, then output == u[1]\u[2]:
  note: (u[2]!=0) is true then returns 1
  note: and finally, the expression is: (u[1] \ u[2]) * 1 = u[1] \ u[2]
  In1 : Inport
  In2 : Inport  Port=2
  Fcn : Fcn  Expr=u[1]/(u[2]+(u[2]==0))*(u[2]!=0)
  Mux : Mux  Inputs=2
  Out1 : Outport
  wires:
  Mux/1 -> Fcn/1
  In1/1 -> Mux/1
  Fcn/1 -> Out1/1
  In2/1 -> Mux/2

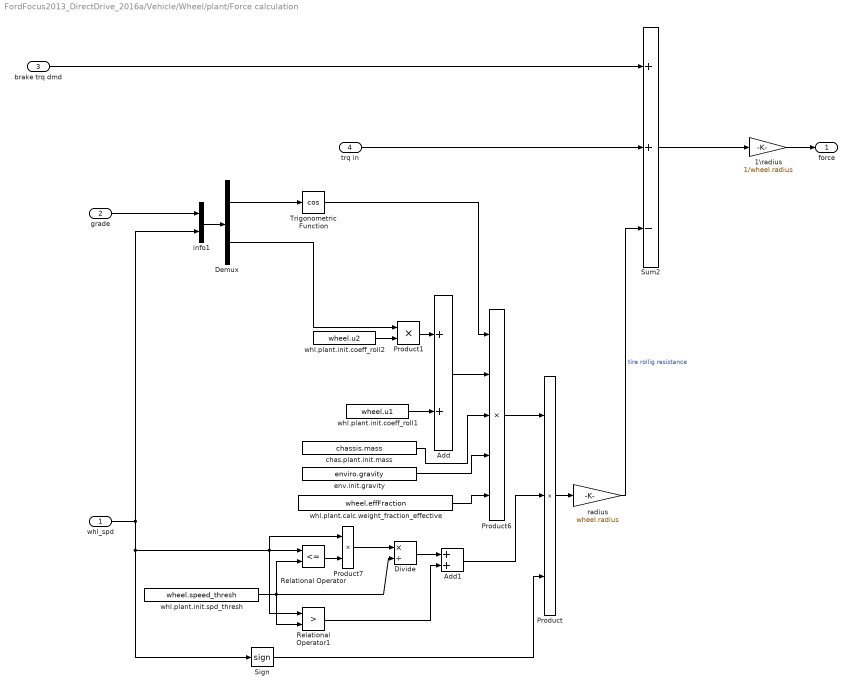
== system FordFocus2013_DirectDrive_2016a/Vehicle/Wheel/plant/Force calculation ==
  whl_spd : Inport
  grade : Inport  Port=2
  brake trq dmd : Inport  Port=3
  trq in : Inport  Port=4
  "1\\radius " : Gain  Gain=1/wheel.radius  SaturateOnIntegerOverflow=on  OutDataTypeStr=Inherit: Same as input  ParamDataTypeStr=Inherit: Same as input
  Add : Sum  Inputs=2
  Add1 : Sum
  Demux : Demux  Outputs=2
  Divide : Product  Inputs=*/
  Product : Product  Inputs=3  SaturateOnIntegerOverflow=on  InputSameDT=on  OutDataTypeStr=Inherit: Same as first input
  Product1 : Product  RndMeth=Zero
  Product6 : Product  Inputs=5  RndMeth=Zero
  Product7 : Product  RndMeth=Zero
  Relational Operator : RelationalOperator  Operator=<=  InputSameDT=on
  Relational Operator1 : RelationalOperator  Operator=>  InputSameDT=on
  Sign : Signum
  Sum2 : Sum  Inputs=++-  SaturateOnIntegerOverflow=on  InputSameDT=on  OutDataTypeStr=Inherit: Same as first input
  Trigonometric Function : Trigonometry  Operator=cos
  chas.plant.init.mass : Constant  Value=chassis.mass
  env.init.gravity : Constant  Value=enviro.gravity
  info1 : Mux  Inputs=2
  radius : Gain  Gain=wheel.radius  SaturateOnIntegerOverflow=on  OutDataTypeStr=Inherit: Same as input  ParamDataTypeStr=Inherit: Same as input
  whl.plant.calc.weight_fraction_effective : Constant  Value=wheel.effFraction
  whl.plant.init.coeff_roll1 : Constant  Value=wheel.u1
  whl.plant.init.coeff_roll2 : Constant  Value=wheel.u2
  whl.plant.init.spd_thresh : Constant  Value=wheel.speed_thresh
  force : Outport
  wires:
  Add1/1 -> Product/2
  Relational Operator1/1 -> Add1/2
  Divide/1 -> Add1/1
  Product7/1 -> Divide/1
  Relational Operator/1 -> Product7/2
  whl.plant.init.spd_thresh/1 -> Relational Operator1/2, Divide/2, Relational Operator/2
  Product6/1 -> Product/1
  Demux/1 -> Trigonometric Function/1
  Trigonometric Function/1 -> Product6/1
  whl.plant.calc.weight_fraction_effective/1 -> Product6/5
  env.init.gravity/1 -> Product6/4
  chas.plant.init.mass/1 -> Product6/3
  Add/1 -> Product6/2
  Product1/1 -> Add/1
  Demux/2 -> Product1/1
  whl.plant.init.coeff_roll2/1 -> Product1/2
  whl_spd/1 -> Relational Operator1/1, Product7/1, Relational Operator/1, Sign/1, info1/2
  radius/1 -> Sum2/3  "tire rollig resistance"
  trq in/1 -> Sum2/2
  info1/1 -> Demux/1
  grade/1 -> info1/1
  Sign/1 -> Product/3
  Product/1 -> radius/1
  brake trq dmd/1 -> Sum2/1
  "1\\radius "/1 -> force/1
  Sum2/1 -> "1\\radius "/1
  whl.plant.init.coeff_roll1/1 -> Add/2

== system FordFocus2013_DirectDrive_2016a/Vehicle/Wheel/plant/Mass calculation ==
  inertia in : Inport
  1\radius^2 : Gain  Gain=1/wheel.radius^2  SaturateOnIntegerOverflow=on  OutDataTypeStr=Inherit: Same as input  ParamDataTypeStr=Inherit: Same as input
  Sum6 : Sum  SaturateOnIntegerOverflow=on  InputSameDT=on  OutDataTypeStr=Inherit: Same as first input
  wheel inertia : Constant  Value=wheel.inertia
  Mass : Outport
  wires:
  wheel inertia/1 -> Sum6/1
  Sum6/1 -> 1\radius^2/1
  1\radius^2/1 -> Mass/1
  inertia in/1 -> Sum6/2

== system FordFocus2013_DirectDrive_2016a/Vehicle/ESS1/plant/ess_plant_soc_calculation/non-zero division1 ==
  note: original idea from Phil Sharer - ANL
      | original formula: u[1]/(u[2]+eps)*(u[2]!=0)
      | changes done by Gerald ZINI (dgey) - ANL (05/02/2001)
  note: (u[2]==0) is true then returns 1, thus (u[2]+(u[2]==0)) is equal to 0+1=1
  note: if u[2] == 0, then output == 0:
  note: (u[2]!=0) is false then returns 0
  note: and finally, the expression is: (u[1] / 1) * 0 = 0
  note: (u[2]==0) is false then returns 0, thus (u[2]+(u[2]==0)) is equal to u[2]+0=u[2]
  note: if u[2] != 0, then output == u[1]/u[2]:
  note: (u[2]!=0) is true then returns 1
  note: and finally, the expression is: (u[1] / u[2]) * 1 = u[1] / u[2]
  In1 : Inport
  In2 : Inport  Port=2
  Fcn : Fcn  Expr=u[1]/(u[2]+(u[2]==0))*(u[2]!=0)
  Mux : Mux  Inputs=2
  Out1 : Outport
  wires:
  Mux/1 -> Fcn/1
  In1/1 -> Mux/1
  Fcn/1 -> Out1/1
  In2/1 -> Mux/2

== system FordFocus2013_DirectDrive_2016a/Vehicle/Final Drive/plant/Torque calculation/non-zero division1 ==
  note: (u[2]==0) is true then returns 1, thus (u[2]+(u[2]==0)) is equal to 0+1=1
  note: if u[2] == 0, then output == 0:
  note: (u[2]!=0) is false then returns 0
  note: and finally, the expression is: (u[1] \ 1) * 0 = 0
  note: (u[2]==0) is false then returns 0, thus (u[2]+(u[2]==0)) is equal to u[2]+0=u[2]
  note: if u[2] != 0, then output == u[1]\u[2]:
  note: (u[2]!=0) is true then returns 1
  note: and finally, the expression is: (u[1] \ u[2]) * 1 = u[1] \ u[2]
  In1 : Inport
  In2 : Inport  Port=2
  Fcn : Fcn  Expr=u[1]/(u[2]+(u[2]==0))*(u[2]!=0)
  Mux : Mux  Inputs=2
  Out1 : Outport
  wires:
  Mux/1 -> Fcn/1
  In1/1 -> Mux/1
  Fcn/1 -> Out1/1
  In2/1 -> Mux/2

== system FordFocus2013_DirectDrive_2016a/Vehicle/Motor/motor/Motor Efficiency/non-zero division1 ==
  note: (u[2]==0) is true then returns 1, thus (u[2]+(u[2]==0)) is equal to 0+1=1
  note: if u[2] == 0, then output == 0:
  note: (u[2]!=0) is false then returns 0
  note: and finally, the expression is: (u[1] \ 1) * 0 = 0
  note: (u[2]==0) is false then returns 0, thus (u[2]+(u[2]==0)) is equal to u[2]+0=u[2]
  note: if u[2] != 0, then output == u[1]\u[2]:
  note: (u[2]!=0) is true then returns 1
  note: and finally, the expression is: (u[1] \ u[2]) * 1 = u[1] \ u[2]
  In1 : Inport
  In2 : Inport  Port=2
  Fcn : Fcn  Expr=u[1]/(u[2]+(u[2]==0))*(u[2]!=0)
  Mux : Mux  Inputs=2
  Out1 : Outport
  wires:
  Mux/1 -> Fcn/1
  In1/1 -> Mux/1
  Fcn/1 -> Out1/1
  In2/1 -> Mux/2
